simulink model "unit1"  (R2020a)
settings: Solver=VariableStepAuto  StartTime=0.0  StopTime=10.0  RelTol=1e-3
settings Model: Creator=fsepcke  LastModifiedBy=fsepcke

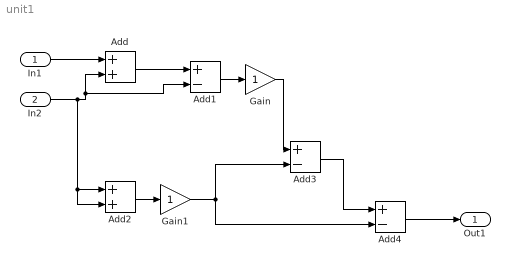
== system unit1 ==
  In1 : Inport
  In2 : Inport  Port=2
  Add : Sum
  Add1 : Sum  Inputs=+-
  Add2 : Sum
  Add3 : Sum  Inputs=+-
  Add4 : Sum  Inputs=+-
  Gain : Gain
  Gain1 : Gain
  Out1 : Outport
  wires:
  Add/1 -> Add1/1
  In1/1 -> Add/1
  In2/1 -> Add2/2, Add2/1, Add1/2, Add/2
  Add1/1 -> Gain/1
  Gain/1 -> Add3/1
  Add2/1 -> Gain1/1
  Add3/1 -> Add4/1
  Add4/1 -> Out1/1
  Gain1/1 -> Add3/2, Add4/2
